simulink model "MotorCrap"  (R2017a)
settings: Solver=ode3  StartTime=0.0  StopTime=10.0  FixedStep=0.002  RelTol=1e-3
libraries: stellaris_lp_lib x17, simulink x4, dspswit3 x3, simulink_extras x1
settings Model: ExtModeTrigDuration=2  Creator=peselnikmg  LastModifiedBy=cwisnew
settings DataIOCC: LimitDataPoints=on  SaveFormat=Array  SignalLoggingSaveFormat=ModelDataLogs
settings OptimizationCC: PassReuseOutputArgsAs=Individual arguments  ExpressionDepthLimit=2147483647  MaxStackSize=64
settings DebuggingCC: ParameterTunabilityLossMsg=error  StateNameClashWarn=warning  SFUnexpectedBacktrackingDiag=warning  SFNoUnconditionalDefaultTransitionDiag=warning  SFExecutionAtInitializationDiag=none
settings HardwareCC: ProdBitPerPointer=32  ProdBitPerSizeT=32  ProdBitPerPtrDiffT=32  ProdLargestAtomicInteger=Long  ProdLargestAtomicFloat=Double  ProdWordSize=32  ProdHWDeviceType=ARM Compatible->ARM Cortex
settings ModelReferenceCC: PropagateSignalLabelsOutOfModel=off
settings SFSimCC: MATLABDynamicMemAlloc=off
settings RTWCC: SystemTargetFile=ert.tlc  HardwareBoard=Tiva TM4C123G Launchpad  TLCOptions=-aInlineSetEventsForThisBaseRateFcn=TLC_FALSE -aSuppressMultiTaskScheduler=TLC_FALSE -aRateBasedStepFcn=1  TemplateMakefile=ert_default_tmf  Description=Embedded Coder  GenerateReport=on  RTWVerbose=off  Toolchain=Texas Instruments Code Composer Studio (Tiva)  IncludeHyperlinkInReport=on  LaunchReport=on  GenerateTraceInfo=on  GenerateTraceReport=on  GenerateTraceReportSl=on  GenerateTraceReportSf=on  GenerateTraceReportEml=on
settings CodeAppCC: ForceParamTrailComments=on  IgnoreCustomStorageClasses=off  OperatorAnnotations=on  SimulinkDataObjDesc=on  SFDataObjDesc=on  MATLABFcnDesc=on  CustomSymbolStrType=$N$R$M  InsertBlockDesc=on  MATLABSourceComments=on  InternalIdentifier=Classic
settings ConfigComp: CovMetricSettings=dw  CovHtmlReporting=on  CovSaveCumulativeToWorkspaceVar=on  CovSaveSingleToWorkspaceVar=on  CovExternalEMLEnable=off

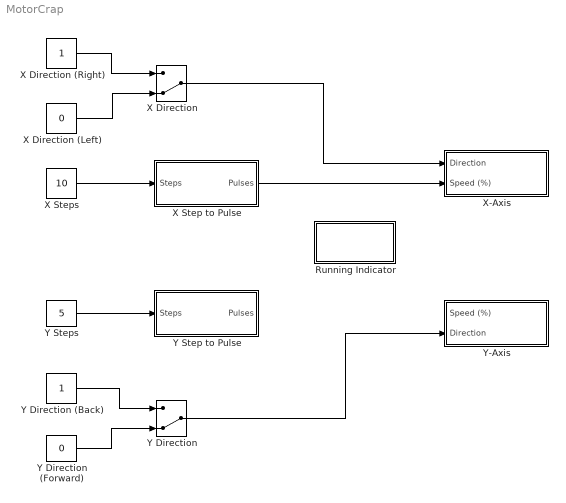
== system MotorCrap ==
  Running Indicator : Subsystem
  X Direction : ManualSwitch  CurrentSetting=0
  X Direction (Left) : Constant  Value=0  OutDataTypeStr=uint8
  X Direction (Right) : Constant  OutDataTypeStr=uint8
  X Step to Pulse : Subsystem  TreatAsAtomicUnit=on
  X Steps : Constant  Value=10  OutDataTypeStr=single
  X-Axis : Subsystem
  Y Direction : ManualSwitch  CurrentSetting=0
  Y Direction (Back) : Constant  OutDataTypeStr=uint8
  Y Direction (Forward) : Constant  Value=0  OutDataTypeStr=uint8
  Y Step to Pulse : Subsystem  TreatAsAtomicUnit=on
  Y Steps : Constant  Value=5  OutDataTypeStr=single
  Y-Axis : Subsystem
  wires:
  Y Direction (Back)/1 -> Y Direction/1
  Y Direction (Forward)/1 -> Y Direction/2
  Y Direction/1 -> Y-Axis/2(Direction)
  X Direction (Right)/1 -> X Direction/1
  X Direction (Left)/1 -> X Direction/2
  X Direction/1 -> X-Axis/1(Direction)
  Y Steps/1 -> Y Step to Pulse/1(Steps)
  ? -> Y-Axis/1(Speed (%))
  X Step to Pulse/1(Pulses) -> X-Axis/2(Speed (%))
  X Steps/1 -> X Step to Pulse/1(Steps)

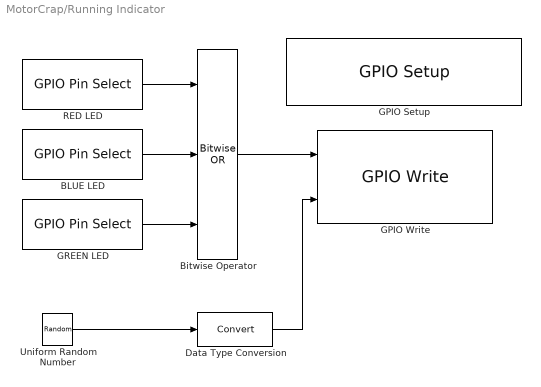
== system MotorCrap/Running Indicator ==
  BLUE LED : stellaris_lp_lib/GPIO/GPIO Pin Select  GPIO_PIN_X=GPIO_PIN_2
      settings: SourceProductName=Run on Stellaris LaunchPad
  Bitwise Operator : simulink/Logic and Bit Operations/Bitwise Operator  logicop=OR  UseBitMask=off  NumInputPorts=3  BitMask=bin2dec('11011001')  BitMaskRealWorld=Stored Integer
  Data Type Conversion : DataTypeConversion
  GPIO Setup : stellaris_lp_lib/GPIO/GPIO Setup  GPIO_PORTX_BASE=GPIO_PORTF_BASE  PinsOutput_0=Input  PinsOutput_1=Output  PinsOutput_2=Output  PinsOutput_3=Output  PinsOutput_4=Input  PinsOutput_5=Input  PinsOutput_6=Input  PinsOutput_7=Input
      settings: SourceProductName=Run on Stellaris LaunchPad
  GPIO Write : stellaris_lp_lib/GPIO/GPIO Write  GPIO_PORTX_BASE=GPIO_PORTF_BASE  SampleTime=-1
      settings: SourceProductName=Run on Stellaris LaunchPad
  GREEN LED : stellaris_lp_lib/GPIO/GPIO Pin Select  GPIO_PIN_X=GPIO_PIN_3
      settings: SourceProductName=Run on Stellaris LaunchPad
  RED LED : stellaris_lp_lib/GPIO/GPIO Pin Select  GPIO_PIN_X=GPIO_PIN_1
      settings: SourceProductName=Run on Stellaris LaunchPad
  Uniform Random Number : UniformRandomNumber  Minimum=0  Maximum=2  SampleTime=0.2
  wires:
  BLUE LED/1 -> Bitwise Operator/2
  RED LED/1 -> Bitwise Operator/1
  GREEN LED/1 -> Bitwise Operator/3
  Bitwise Operator/1 -> GPIO Write/1
  Uniform Random Number/1 -> Data Type Conversion/1
  Data Type Conversion/1 -> GPIO Write/2

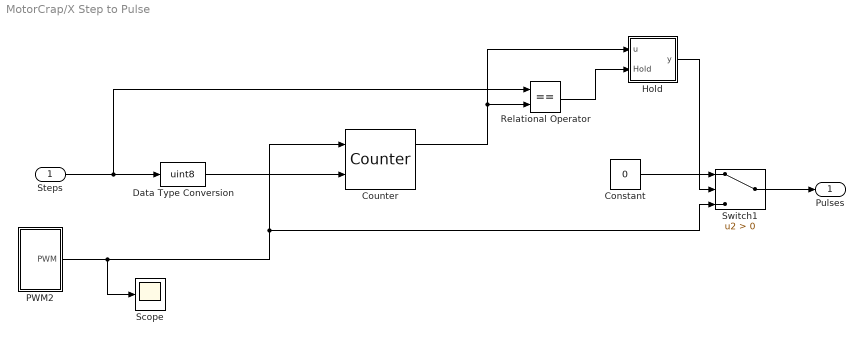
== system MotorCrap/X Step to Pulse ==
  Steps : Inport
  Constant : Constant  Value=0  OutDataTypeStr=single
  Counter : dspswit3/Counter  Direction=Up  CountEvent=Rising edge  CounterSize=Specify via input port  MaxCount=255  InitialCount=0  Output=Count and Hit  HitValue=2  ResetInput=off  SamplesPerFrame=1  Ts=1  CntDtype=single  HitDtype=Logical
  Data Type Conversion : DataTypeConversion  OutDataTypeStr=uint8
  Hold : Subsystem  TreatAsAtomicUnit=on
  PWM2 : Subsystem
  Relational Operator : RelationalOperator  Operator===  OutDataTypeStr=boolean  RndMeth=Simplest
  Scope : Scope
  Switch1 : Switch  Criteria=u2 > Threshold
  Pulses : Outport
  wires:
  Steps/1 -> Relational Operator/1, Data Type Conversion/1
  Data Type Conversion/1 -> Counter/2
  Relational Operator/1 -> Hold/2(Hold)
  Switch1/1 -> Pulses/1
  Hold/1(y) -> Switch1/2
  Counter/1 -> Hold/1(u), Relational Operator/2
  Constant/1 -> Switch1/1
  PWM2/1(PWM) -> Scope/1, Counter/1, Switch1/3

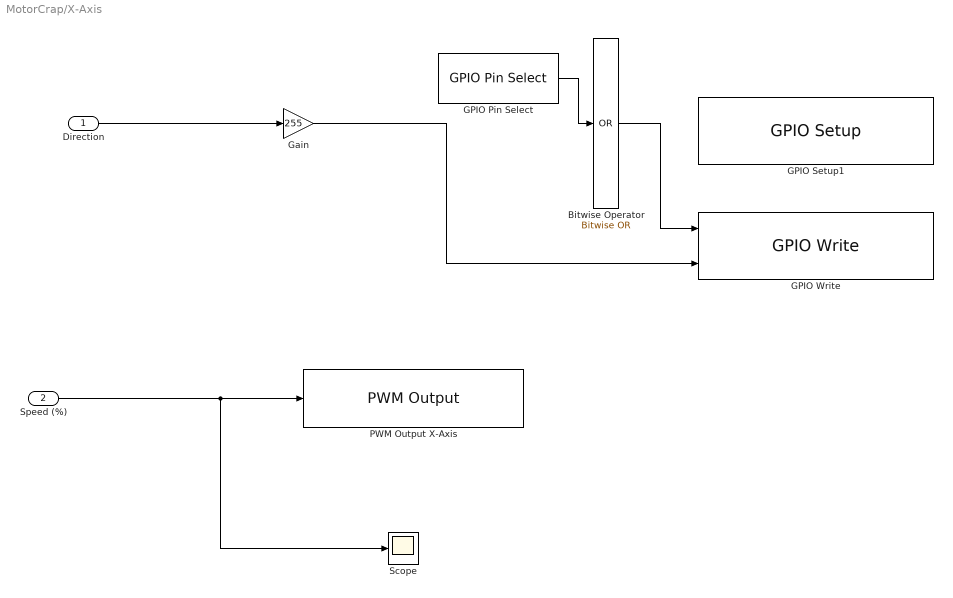
== system MotorCrap/X-Axis ==
  Direction : Inport  OutDataTypeStr=uint8
  Speed (%) : Inport  Port=2  OutDataTypeStr=single
  Bitwise Operator : simulink/Logic and Bit Operations/Bitwise Operator  logicop=OR  UseBitMask=off  BitMask=bin2dec('11011001')  BitMaskRealWorld=Real World Value
  GPIO Pin Select : stellaris_lp_lib/GPIO/GPIO Pin Select  GPIO_PIN_X=GPIO_PIN_5
      settings: SourceProductName=Run on Stellaris LaunchPad
  GPIO Setup1 : stellaris_lp_lib/GPIO/GPIO Setup  GPIO_PORTX_BASE=GPIO_PORTA_BASE  PinsOutput_0=Unused  PinsOutput_1=Unused  PinsOutput_2=Output  PinsOutput_3=Unused  PinsOutput_4=Unused  PinsOutput_5=Unused  PinsOutput_6=Unused  PinsOutput_7=Unused
      settings: SourceProductName=Run on Stellaris LaunchPad
  GPIO Write : stellaris_lp_lib/GPIO/GPIO Write  GPIO_PORTX_BASE=GPIO_PORTC_BASE  SampleTime=-1
      settings: SourceProductName=Run on Stellaris LaunchPad
  Gain : Gain  Gain=255  ParamDataTypeStr=uint8  OutDataTypeStr=uint8
  PWM Output X-Axis : stellaris_lp_lib/PWM/PWM Output  ch="3    PC6"  invert=off  freq=100  sample_time=-1
      settings: SourceProductName=Run on Stellaris LaunchPad
  Scope : Scope
  wires:
  Direction/1 -> Gain/1
  GPIO Pin Select/1 -> Bitwise Operator/1
  Bitwise Operator/1 -> GPIO Write/1
  Gain/1 -> GPIO Write/2
  Speed (%)/1 -> Scope/1, PWM Output X-Axis/1

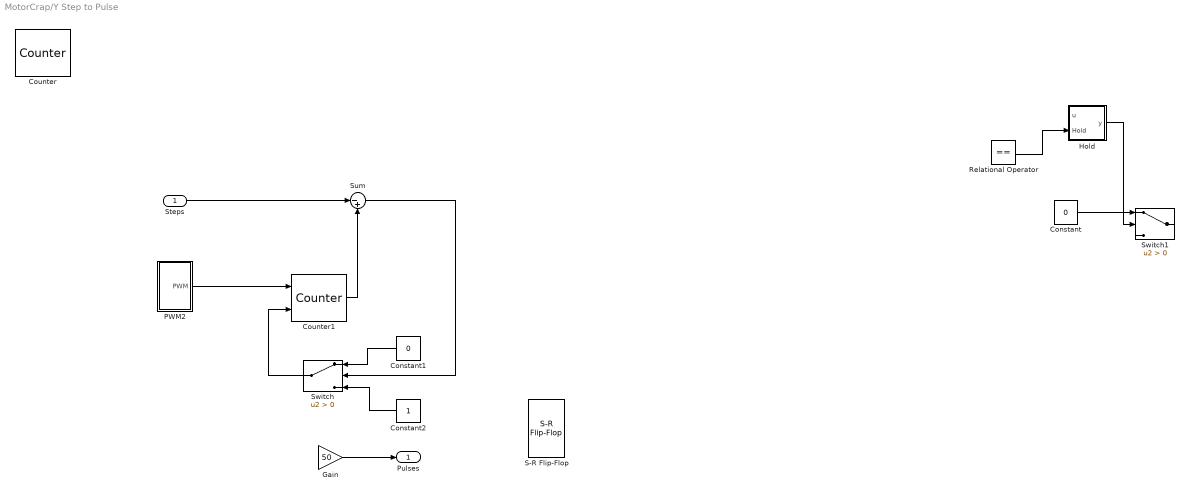
== system MotorCrap/Y Step to Pulse ==
  Steps : Inport
  Constant : Constant  Value=0  OutDataTypeStr=single
  Constant1 : Constant  Value=0
  Constant2 : Constant
  Counter : dspswit3/Counter  Direction=Up  CountEvent=Rising edge  CounterSize=Specify via input port  MaxCount=255  InitialCount=0  Output=Count and Hit  HitValue=2  ResetInput=off  SamplesPerFrame=1  Ts=1  CntDtype=single  HitDtype=Logical
  Counter1 : dspswit3/Counter  Direction=Up  CountEvent=Rising edge  CounterSize=User defined  MaxCount=255  InitialCount=0  Output=Count  HitValue=32  ResetInput=on  SamplesPerFrame=1  Ts=1  CntDtype=double  HitDtype=Logical
  Gain : Gain  Gain=50
  Hold : Subsystem  TreatAsAtomicUnit=on
  PWM2 : Subsystem
  Relational Operator : RelationalOperator  Operator===  OutDataTypeStr=boolean  RndMeth=Simplest
  S-R Flip-Flop : simulink_extras/Flip Flops/S-R Flip-Flop  initial_condition=0
  Sum : Sum  Inputs=|-+
  Switch : Switch  Criteria=u2 > Threshold
  Switch1 : Switch  Criteria=u2 > Threshold
  Pulses : Outport
  wires:
  Steps/1 -> Sum/1
  PWM2/1(PWM) -> Counter1/1
  Counter1/1 -> Sum/2
  Constant/1 -> Switch1/1
  Hold/1(y) -> Switch1/2
  ? -> Switch1/3
  ? -> Relational Operator/1
  Relational Operator/1 -> Hold/2(Hold)
  ? -> Hold/1(u)
  ? -> Relational Operator/2
  Switch/1 -> Counter1/2
  Sum/1 -> Switch/2
  Constant1/1 -> Switch/1
  Constant2/1 -> Switch/3
  Gain/1 -> Pulses/1
  ? -> Gain/1

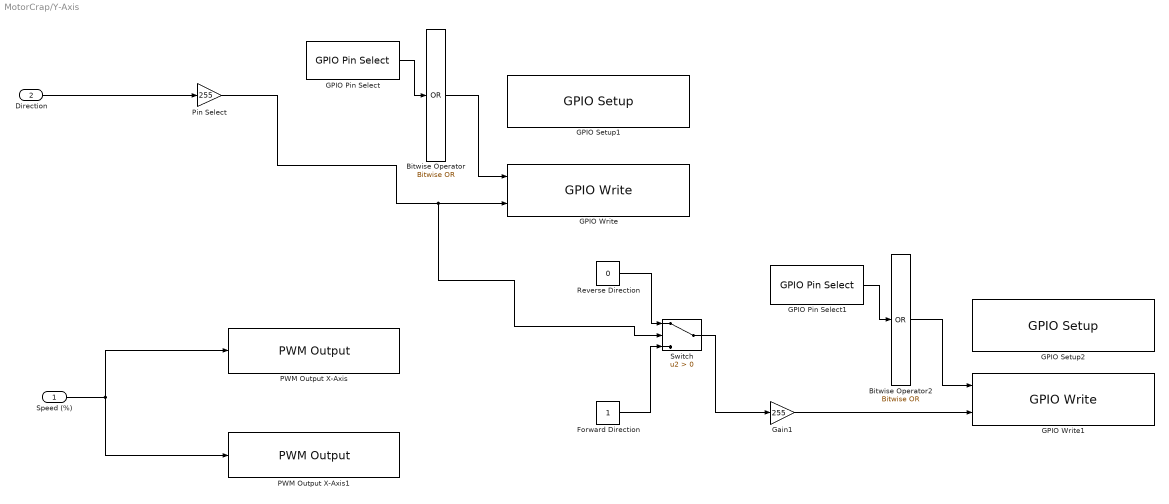
== system MotorCrap/Y-Axis ==
  Speed (%) : Inport  OutDataTypeStr=single
  Direction : Inport  Port=2  OutDataTypeStr=uint8
  Bitwise Operator : simulink/Logic and Bit Operations/Bitwise Operator  logicop=OR  UseBitMask=off  BitMask=bin2dec('11011001')  BitMaskRealWorld=Stored Integer
  Bitwise Operator2 : simulink/Logic and Bit Operations/Bitwise Operator  logicop=OR  UseBitMask=off  BitMask=bin2dec('11011001')  BitMaskRealWorld=Stored Integer
  Forward Direction : Constant  OutDataTypeStr=uint8
  GPIO Pin Select : stellaris_lp_lib/GPIO/GPIO Pin Select  GPIO_PIN_X=GPIO_PIN_0
      settings: SourceProductName=Run on Stellaris LaunchPad
  GPIO Pin Select1 : stellaris_lp_lib/GPIO/GPIO Pin Select  GPIO_PIN_X=GPIO_PIN_1
      settings: SourceProductName=Run on Stellaris LaunchPad
  GPIO Setup1 : stellaris_lp_lib/GPIO/GPIO Setup  GPIO_PORTX_BASE=GPIO_PORTB_BASE  PinsOutput_0=Output  PinsOutput_1=Unused  PinsOutput_2=Unused  PinsOutput_3=Unused  PinsOutput_4=Unused  PinsOutput_5=Unused  PinsOutput_6=Unused  PinsOutput_7=Unused
      settings: SourceProductName=Run on Stellaris LaunchPad
  GPIO Setup2 : stellaris_lp_lib/GPIO/GPIO Setup  GPIO_PORTX_BASE=GPIO_PORTB_BASE  PinsOutput_0=Unused  PinsOutput_1=Output  PinsOutput_2=Unused  PinsOutput_3=Unused  PinsOutput_4=Unused  PinsOutput_5=Unused  PinsOutput_6=Unused  PinsOutput_7=Unused
      settings: SourceProductName=Run on Stellaris LaunchPad
  GPIO Write : stellaris_lp_lib/GPIO/GPIO Write  GPIO_PORTX_BASE=GPIO_PORTB_BASE  SampleTime=-1
      settings: SourceProductName=Run on Stellaris LaunchPad
  GPIO Write1 : stellaris_lp_lib/GPIO/GPIO Write  GPIO_PORTX_BASE=GPIO_PORTB_BASE  SampleTime=-1
      settings: SourceProductName=Run on Stellaris LaunchPad
  Gain1 : Gain  Gain=255  ParamDataTypeStr=uint8  OutDataTypeStr=uint8
  PWM Output X-Axis : stellaris_lp_lib/PWM/PWM Output  ch="2    PC5"  invert=off  freq=100  sample_time=-1
      settings: SourceProductName=Run on Stellaris LaunchPad
  PWM Output X-Axis1 : stellaris_lp_lib/PWM/PWM Output  ch="3    PC6"  invert=off  freq=100  sample_time=-1
      settings: SourceProductName=Run on Stellaris LaunchPad
  Pin Select : Gain  Gain=255  ParamDataTypeStr=uint8  OutDataTypeStr=uint8
  Reverse Direction : Constant  Value=0  OutDataTypeStr=uint8
  Switch : Switch  Criteria=u2 > Threshold  OutDataTypeStr=uint8
  wires:
  Direction/1 -> Pin Select/1
  GPIO Pin Select/1 -> Bitwise Operator/1
  Bitwise Operator/1 -> GPIO Write/1
  GPIO Pin Select1/1 -> Bitwise Operator2/1
  Bitwise Operator2/1 -> GPIO Write1/1
  Switch/1 -> Gain1/1
  Gain1/1 -> GPIO Write1/2
  Reverse Direction/1 -> Switch/1
  Forward Direction/1 -> Switch/3
  Pin Select/1 -> Switch/2, GPIO Write/2
  Speed (%)/1 -> PWM Output X-Axis/1, PWM Output X-Axis1/1

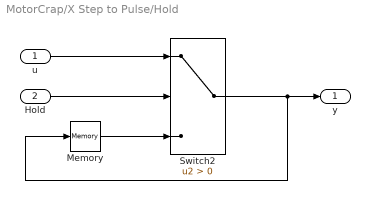
== system MotorCrap/X Step to Pulse/Hold ==
  u : Inport  OutDataTypeStr=single
  Hold : Inport  Port=2  OutDataTypeStr=boolean
  Memory : Memory
  Switch2 : Switch  Criteria=u2 > Threshold  OutDataTypeStr=single
  y : Outport  OutDataTypeStr=single
  wires:
  u/1 -> Switch2/1
  Switch2/1 -> Memory/1, y/1
  Memory/1 -> Switch2/3
  Hold/1 -> Switch2/2

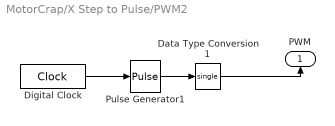
== system MotorCrap/X Step to Pulse/PWM2 ==
  Data Type Conversion1 : DataTypeConversion  OutDataTypeStr=single
  Digital Clock : DigitalClock  SampleTime=-1
  Pulse Generator1 : DiscretePulseGenerator  PulseType=Time based  TimeSource=Use external signal  Amplitude=50  Period=0.1  PulseWidth=98
  PWM : Outport
  wires:
  Digital Clock/1 -> Pulse Generator1/1
  Pulse Generator1/1 -> Data Type Conversion1/1
  Data Type Conversion1/1 -> PWM/1

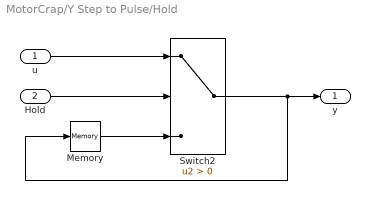
== system MotorCrap/Y Step to Pulse/Hold ==
  u : Inport  OutDataTypeStr=single
  Hold : Inport  Port=2  OutDataTypeStr=boolean
  Memory : Memory
  Switch2 : Switch  Criteria=u2 > Threshold  OutDataTypeStr=single
  y : Outport  OutDataTypeStr=single
  wires:
  u/1 -> Switch2/1
  Switch2/1 -> Memory/1, y/1
  Memory/1 -> Switch2/3
  Hold/1 -> Switch2/2

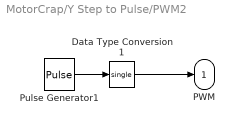
== system MotorCrap/Y Step to Pulse/PWM2 ==
  Data Type Conversion1 : DataTypeConversion  OutDataTypeStr=single
  Pulse Generator1 : DiscretePulseGenerator  PulseType=Time based  Period=0.00167  PulseWidth=50
  PWM : Outport
  wires:
  Pulse Generator1/1 -> Data Type Conversion1/1
  Data Type Conversion1/1 -> PWM/1
